simulink model "quartermodel"  (R2018b)
settings: Solver=VariableStepAuto  StartTime=0.0  StopTime=10.0  RelTol=1e-3
PreLoadFcn:
  | initModel;
PostLoadFcn:
  | load('baseVehicleData');
values from neighbouring files (symbols this model uses):
  g = 9.81    [baseVehicleData.mat]    (also in initModel.m; initModelQuarter.m)
  ks = 20000    [baseVehicleData.mat]    (also in initModel.m; initModelQuarter.m)
  kT = 140000    [baseVehicleData.mat]    (also in initModel.m; initModelQuarter.m)
  m1 = 250    [baseVehicleData.mat]    (also in initModel.m; initModelQuarter.m)
  m2 = 20    [baseVehicleData.mat]    (also in initModel.m; initModelQuarter.m)
  x0 = 0.2    [baseVehicleData.mat]    (also in initModelQuarter.m)
CloseFcn:
  | willSave;
settings Model: Creator=Jamie  LastModifiedBy=jubja

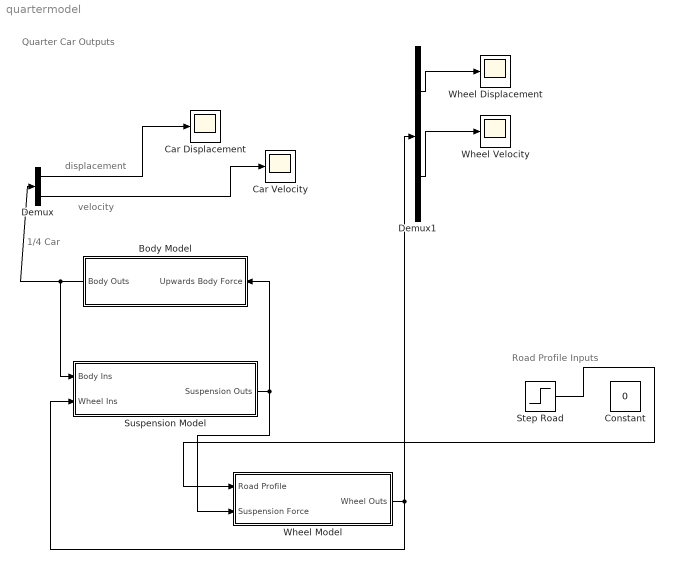
== system quartermodel ==
  note: 1/4 Car
  note: Quarter Car Outputs
  note: Road Profile Inputs
  note: velocity
  note: displacement
  Body Model : Subsystem
  Car Displacement : Scope
  Car Velocity : Scope
  Constant : Constant  Value=0
  Demux : Demux  Outputs=2
  Demux1 : Demux  Outputs=2
  Step Road : Step  Time=3  After=0.1  SampleTime=0
  Suspension Model : Subsystem
  Wheel Displacement : Scope
  Wheel Model : Subsystem
  Wheel Velocity : Scope
  wires:
  Body Model/1(Body Outs) -> Demux/1, Suspension Model/1(Body Ins)
  Suspension Model/1(Suspension Outs) -> Body Model/1(Upwards Body Force), Wheel Model/2(Suspension Force)
  Demux/1 -> Car Displacement/1
  Demux/2 -> Car Velocity/1
  Step Road/1 -> Wheel Model/1(Road Profile)
  Wheel Model/1(Wheel Outs) -> Demux1/1, Suspension Model/2(Wheel Ins)
  Demux1/2 -> Wheel Velocity/1
  Demux1/1 -> Wheel Displacement/1

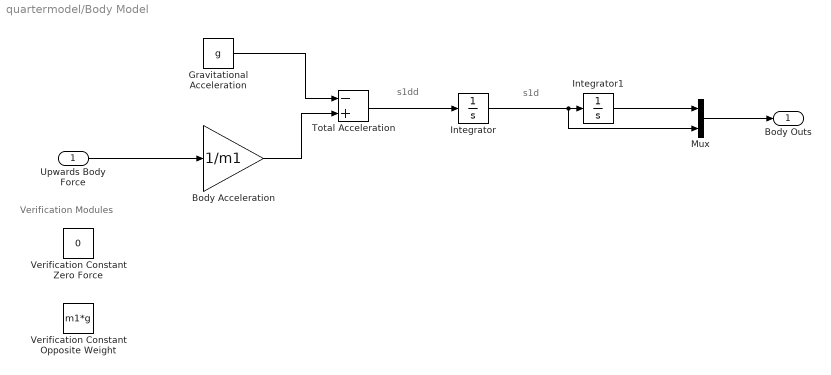
== system quartermodel/Body Model ==
  note: Verification Modules
  note: s1d
  note: s1dd
  Upwards Body Force : Inport
  Body Acceleration : Gain  Gain=1/m1
  Gravitational Acceleration : Constant  Value=g  mask{g=g}
      mask prompts: g "Gravitational Acceleration"
  Integrator : Integrator
  Integrator1 : Integrator
  Mux : Mux  Inputs=2
  Total Acceleration : Sum  Inputs=-+
  Verification Constant Opposite Weight : Constant  Value=m1*g
  Verification Constant Zero Force : Constant  Value=0
  Body Outs : Outport
  wires:
  Integrator1/1 -> Mux/1
  Total Acceleration/1 -> Integrator/1
  Body Acceleration/1 -> Total Acceleration/2
  Integrator/1 -> Mux/2, Integrator1/1
  Mux/1 -> Body Outs/1
  Gravitational Acceleration/1 -> Total Acceleration/1
  Upwards Body Force/1 -> Body Acceleration/1

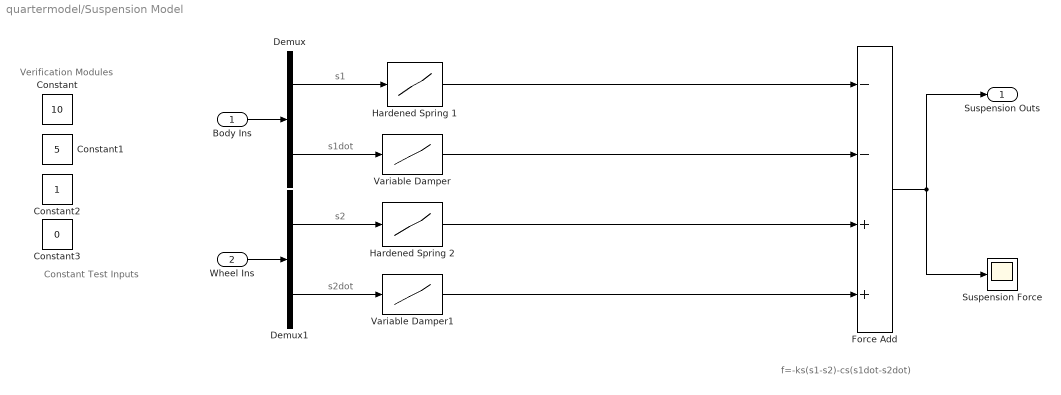
== system quartermodel/Suspension Model ==
  note: Constant Test
      | Inputs
  note: Verification Modules
  note: s2dot
  note: s2
  note: f=-ks(s1-s2)-cs(s1dot-s2dot)
  note: s1dot
  note: s1
  Body Ins : Inport
  Wheel Ins : Inport  Port=2
  Constant : Constant  Value=10
  Constant1 : Constant  Value=5
  Constant2 : Constant
  Constant3 : Constant  Value=0
  Demux : Demux  Outputs=2
  Demux1 : Demux  Outputs=2
  "Force Add " : Sum  Inputs=--++
  Hardened Spring 1 : Lookup_n-D  NumberOfTableDimensions=1  BreakpointsForDimension1=[-2*x0,-x0,x0,2*x0]  Table=[-21*ks*x0,-ks*x0,ks*x0,21*ks*x0]  InternalRulePriority=Speed  RndMeth=Simplest  InputSameDT=on
  Hardened Spring 2 : Lookup_n-D  NumberOfTableDimensions=1  BreakpointsForDimension1=[-2*x0,-x0,x0,2*x0]  Table=[-21*ks*x0,-ks*x0,ks*x0,21*ks*x0]  InternalRulePriority=Speed  RndMeth=Simplest  InputSameDT=on
  Suspension Force : Scope
  Variable Damper : Lookup_n-D  NumberOfTableDimensions=1  BreakpointsForDimension1=[-1,0,1]  Table=[-1200,0,600]  InternalRulePriority=Speed  RndMeth=Simplest  InputSameDT=on
  Variable Damper1 : Lookup_n-D  NumberOfTableDimensions=1  BreakpointsForDimension1=[-1,0,1]  Table=[-1200,0,600]  InternalRulePriority=Speed  RndMeth=Simplest  InputSameDT=on
  Suspension Outs : Outport
  wires:
  Body Ins/1 -> Demux/1
  Wheel Ins/1 -> Demux1/1
  "Force Add "/1 -> Suspension Force/1, Suspension Outs/1
  Hardened Spring 1/1 -> "Force Add "/1
  Variable Damper/1 -> "Force Add "/2
  Hardened Spring 2/1 -> "Force Add "/3
  Variable Damper1/1 -> "Force Add "/4
  Demux1/2 -> Variable Damper1/1
  Demux1/1 -> Hardened Spring 2/1
  Demux/2 -> Variable Damper/1
  Demux/1 -> Hardened Spring 1/1

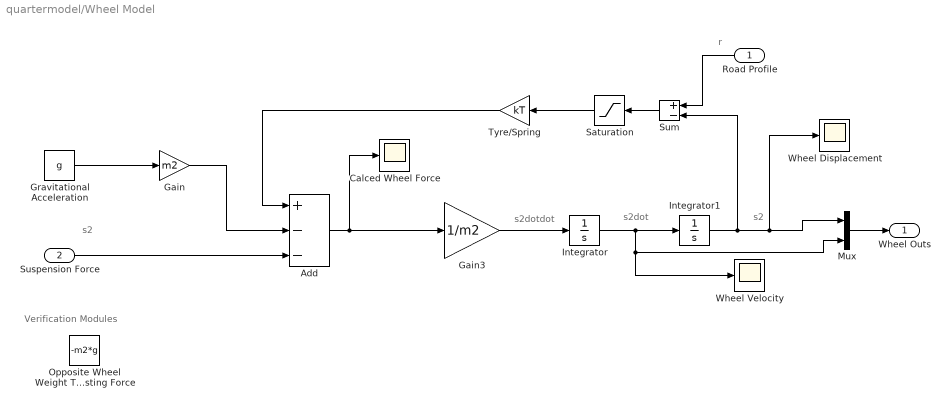
== system quartermodel/Wheel Model ==
  note: s2
  note: s2dot
  note: s2dotdot
  note: r
  note: s2
  note: Verification Modules
  Road Profile : Inport
  Suspension Force : Inport  Port=2
  Add : Sum  Inputs=+--
  Calced Wheel Force : Scope
  Gain : Gain  Gain=m2
  Gain3 : Gain  Gain=1/m2
  Gravitational Acceleration : Constant  Value=g  mask{g=g}
      mask prompts: g "Gravitatioanl Acceleration"
  Integrator : Integrator
  Integrator1 : Integrator
  Mux : Mux  Inputs=2
  Opposite Wheel Weight Testing Force : Constant  Value=-m2*g
  Saturation : Saturate  UpperLimit=inf  LowerLimit=0
  Sum : Sum  Inputs=+-
  "Tyre/Spring " : Gain  Gain=kT
  Wheel Displacement : Scope
  Wheel Velocity : Scope
  Wheel Outs : Outport
  wires:
  Road Profile/1 -> Sum/1
  Gravitational Acceleration/1 -> Gain/1
  Gain3/1 -> Integrator/1
  Integrator/1 -> Wheel Velocity/1, Mux/2, Integrator1/1
  Integrator1/1 -> Sum/2, Wheel Displacement/1, Mux/1
  Mux/1 -> Wheel Outs/1
  Gain/1 -> Add/2
  Suspension Force/1 -> Add/3
  Add/1 -> Gain3/1, Calced Wheel Force/1
  "Tyre/Spring "/1 -> Add/1
  Sum/1 -> Saturation/1
  Saturation/1 -> "Tyre/Spring "/1
